simulink model "Simulare_Hrenciuc_Alexandru_motor_Petrom"  (R2018b)
settings: Solver=FixedStepAuto  StartTime=0.0  StopTime=0.2  FixedStep=0.00001  RelTol=1e-3
libraries: powerlib x19, powerlib_meascontrol x1, simulink x1
settings Model: Creator=alexa  LastModifiedBy=alexa

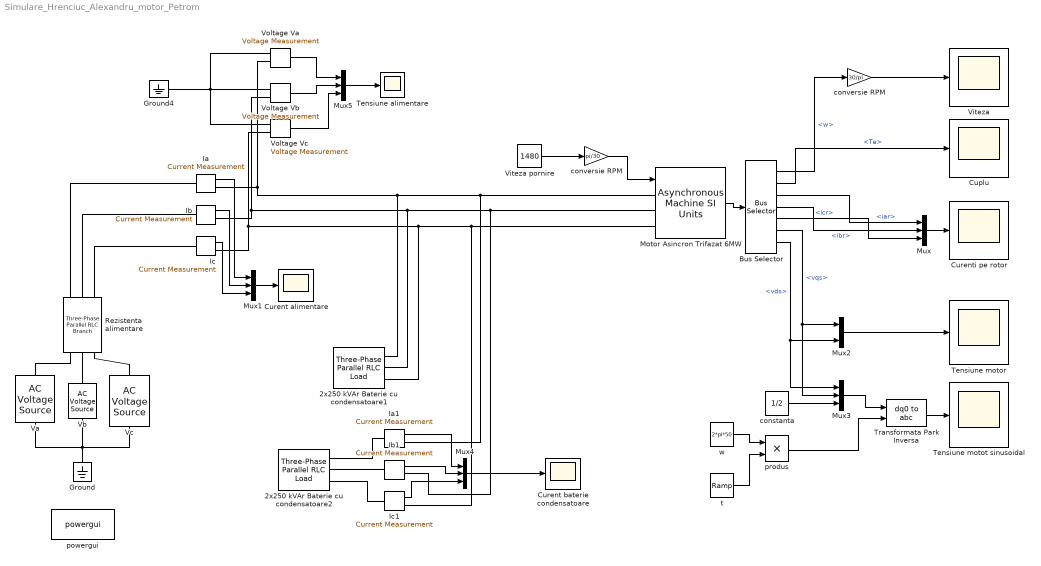
== system Simulare_Hrenciuc_Alexandru_motor_Petrom ==
  2x250 kVAr Baterie cu condensatoare1 : powerlib/Elements/Three-Phase Parallel RLC Load  LConnTagsString=A|B|C  Configuration=Delta  NominalVoltage=6000  Vabc=[1e3 1e3 1e3]  Vabcp=[1e3 1e3 1e3]  NominalFrequency=50  UnbalancedPower=off  ActivePower=0  InductivePower=0  CapacitivePower=5000000  Pabc=[10e3 9e3 11e3]  QLabc=[100 90 110]  QCabc=[100 90 110]  Pabcp=[10e3 9e3 11e3]  QLabcp=[100 90 110]  QCabcp=[100 90 110]  Measurements=Branch currents  LoadType=constant I
  2x250 kVAr Baterie cu condensatoare2 : powerlib/Elements/Three-Phase Parallel RLC Load  LConnTagsString=A|B|C  Configuration=Delta  NominalVoltage=6000  Vabc=[1e3 1e3 1e3]  Vabcp=[1e3 1e3 1e3]  NominalFrequency=50  UnbalancedPower=off  ActivePower=0  InductivePower=0  CapacitivePower=500000  Pabc=[10e3 9e3 11e3]  QLabc=[100 90 110]  QCabc=[100 90 110]  Pabcp=[0 0 0]  QLabcp=[0 0 0]  QCabcp=[1000 900 1100]  Measurements=Branch currents  LoadType=constant I
  Bus Selector : BusSelector  OutputSignals=w,Te,iar,ibr,icr,vqs,vds
  Cuplu : Scope
  Curent alimentare : Scope
  Curent baterie condensatoare : Scope
  Curenti pe rotor : Scope
  Ground : powerlib/Elements/Ground  LConnTagsString=a
  Ground4 : powerlib/Elements/Ground  LConnTagsString=a
  Ia : powerlib/Measurements/Current Measurement  PhasorSimulation=off  OutputType=Magnitude  PSBequivalent=0
  Ia1 : powerlib/Measurements/Current Measurement  PhasorSimulation=off  OutputType=Magnitude  PSBequivalent=0
  Ib : powerlib/Measurements/Current Measurement  PhasorSimulation=off  OutputType=Magnitude  PSBequivalent=0
  Ib1 : powerlib/Measurements/Current Measurement  PhasorSimulation=off  OutputType=Magnitude  PSBequivalent=0
  Ic : powerlib/Measurements/Current Measurement  PhasorSimulation=off  OutputType=Magnitude  PSBequivalent=0
  Ic1 : powerlib/Measurements/Current Measurement  PhasorSimulation=off  OutputType=Magnitude  PSBequivalent=0
  Motor Asincron Trifazat 6MW : powerlib/Machines/Asynchronous Machine SI Units  RotorType=Squirrel-cage  PresetModel=No  MechanicalLoad=Speed w  ShowDetailedParameters=on  ReferenceFrame=Synchronous  Units=SI  MeasurementBus=on  NominalParameters=[6.714e+06 6000 50]  Stator=[0.4 0.00064339]  Rotor=[0.82 0.00064339]  Cage1=[0.4155 0.002066]  Cage2=[0.4168 0.0003495]  Lm=0.0134  Mechanical=[330 0.005879 2]  PolePairs=2  InitialConditions=[0 0 0 0 0 0 0 0]  SimulateSaturation=off  Saturation=[14.03593122, 27.81365428, 53.79336849, 72.68890987, 97.98006896, 148.6815601, 215.7428561, 302.9841135, 428.7778367 ; 230, 322, 414, 460, 506, 552, 598, 644, 690]  LoadFlowParameters=1492000  TsPowergui=0  TsBlock=-1  IterativeModel=Trapezoidal non iterative  IterativeDiscreteModel=Trapezoidal non iterative  Pmec=6714000
  Mux{,1,3..5} (5 alike) : Mux  Inputs=3
  Mux2 : Mux  Inputs=2
  Rezistenta alimentare : powerlib/Elements/Three-Phase Parallel RLC Branch  LConnTagsString=A|B|C  RConnTagsString=A|B|C  BranchType=R  Resistance=0.95  Inductance=1e-3  Capacitance=1e-6  Measurements=None
      settings: SourceProductName=Simscape Power Systems  SourceProductBaseCode=PS
  Tensiune alimentare : Scope
  Tensiune motor : Scope
  Tensiune motot sinusoidal : Scope
  Transformata Park Inversa : powerlib_meascontrol/Transformations/dq0 to abc  Alignment=90 degrees behind phase A axis
  Va : powerlib/Electrical Sources/AC Voltage Source  Amplitude=4899  Phase=0  Frequency=50  SampleTime=0  Measurements=None  BusType=swing  Pref=10e3  Qref=0  Qmin=-inf  Qmax=+inf
  "Vb " : powerlib/Electrical Sources/AC Voltage Source  Amplitude=4899  Phase=-120  Frequency=50  SampleTime=0  Measurements=None  BusType=swing  Pref=10e3  Qref=0  Qmin=-inf  Qmax=+inf
  Vc : powerlib/Electrical Sources/AC Voltage Source  Amplitude=4899  Phase=120  Frequency=50  SampleTime=0  Measurements=None  BusType=swing  Pref=10e3  Qref=0  Qmin=-inf  Qmax=+inf
  Viteza : Scope
  Viteza pornire : Constant  Value=1480
  Voltage Va : powerlib/Measurements/Voltage Measurement  PhasorSimulation=off  OutputType=Complex  PSBequivalent=0
  Voltage Vb : powerlib/Measurements/Voltage Measurement  PhasorSimulation=off  OutputType=Complex  PSBequivalent=0
  Voltage Vc : powerlib/Measurements/Voltage Measurement  PhasorSimulation=off  OutputType=Complex  PSBequivalent=0
  "constanta " : Constant  Value=1/2
  conversie RPM : Gain  Gain=30/pi  SaturateOnIntegerOverflow=on  OutDataTypeStr=Inherit: Same as input  ParamDataTypeStr=Inherit: Same as input
  "conversie RPM " : Gain  Gain=pi/30  SaturateOnIntegerOverflow=on  OutDataTypeStr=Inherit: Same as input  ParamDataTypeStr=Inherit: Same as input
  powergui : powerlib/powergui  Priority=1  SimulationMode=Discrete  SampleTime=50e-6  frequency=50  Iterations=50  frequencyindice=50  Pbase=100e6  ErrMax=1e-4  UnitsV=kV  UnitsW=MW  buscounter=0  FunctionMessages=off  echomessages=off  EnableUseOfTLC=off  CurrentSourceSwitches=off  DisableSnubberDevices=off  DisableRonSwitches=off  DisableVfSwitches=off  DisplayEquations=off  SolverType=Tustin/Backward Euler (TBE)  Interpol=off  ExternalGateDelay=off  methode=off  Ts=100  x0status=blocks  SPID=off  SwTol=0  HookPort=off  RestoreLinks=warning  ResistiveCurrentMeasurement=off  Frange=[0:2:500]  Ylog=off  Xlog=on  ShowGrid=off  save=off  variable=ZData  structure=0  ZoomFFT=off  StartTime=0.0  cycles=1  DisplayStyle=1  fundamental=60  FreqAxis=off  MaxFrequency=1000  frequencyindicesteady=1  RmsSteady=1  display=off
  produs : Product  Inputs=**
  t : simulink/Sources/Ramp  slope=1  start=0  InitialOutput=0
  w : Constant  Value=2*pi*50
  wires:
  conversie RPM/1 -> Viteza/1
  Bus Selector/1 -> conversie RPM/1  "<w>"
  Motor Asincron Trifazat 6MW/1 -> Bus Selector/1
  Mux/1 -> Curenti pe rotor/1
  Ia/1 -> Mux1/1
  Ib/1 -> Mux1/2
  Ic/1 -> Mux1/3
  Mux1/1 -> Curent alimentare/1
  Transformata Park Inversa/1 -> Tensiune motot sinusoidal/1
  w/1 -> produs/1
  t/1 -> produs/2
  produs/1 -> Transformata Park Inversa/2
  Mux3/1 -> Transformata Park Inversa/1
  "constanta "/1 -> Mux3/3
  Mux2/1 -> Tensiune motor/1
  Ia1/1 -> Mux4/1
  Ib1/1 -> Mux4/2
  Ic1/1 -> Mux4/3
  Mux4/1 -> Curent baterie condensatoare/1
  Bus Selector/2 -> Cuplu/1  "<Te>"
  Bus Selector/3 -> Mux/1  "<iar>"
  Bus Selector/4 -> Mux/2  "<ibr>"
  Bus Selector/5 -> Mux/3  "<icr>"
  Bus Selector/6 -> Mux3/2, Mux2/1  "<vqs>"
  Bus Selector/7 -> Mux3/1, Mux2/2  "<vds>"
  Viteza pornire/1 -> "conversie RPM "/1
  "conversie RPM "/1 -> Motor Asincron Trifazat 6MW/1
  Mux5/1 -> Tensiune alimentare/1
  Voltage Va/1 -> Mux5/1
  Voltage Vb/1 -> Mux5/2
  Voltage Vc/1 -> Mux5/3
  connections:
  Va/LConn1 -- "Vb "/LConn1 -- Ground/LConn1 -- Vc/LConn1
  Ib/RConn1 -- Voltage Vb/LConn2 -- Ib1/RConn1 -- Motor Asincron Trifazat 6MW/LConn2 -- 2x250 kVAr Baterie cu condensatoare1/LConn2
  Ic/RConn1 -- Voltage Vc/LConn2 -- Motor Asincron Trifazat 6MW/LConn3 -- Ic1/RConn1 -- 2x250 kVAr Baterie cu condensatoare1/LConn3
  Va/RConn1 -- Rezistenta alimentare/LConn1
  "Vb "/RConn1 -- Rezistenta alimentare/LConn2
  Vc/RConn1 -- Rezistenta alimentare/LConn3
  Rezistenta alimentare/RConn1 -- Ia/LConn1
  Rezistenta alimentare/RConn2 -- Ib/LConn1
  Rezistenta alimentare/RConn3 -- Ic/LConn1
  Ia1/LConn1 -- 2x250 kVAr Baterie cu condensatoare2/LConn1
  Ib1/LConn1 -- 2x250 kVAr Baterie cu condensatoare2/LConn2
  Ic1/LConn1 -- 2x250 kVAr Baterie cu condensatoare2/LConn3
  Ia/RConn1 -- Voltage Va/LConn2 -- Ia1/RConn1 -- Motor Asincron Trifazat 6MW/LConn1 -- 2x250 kVAr Baterie cu condensatoare1/LConn1
  Ground4/LConn1 -- Voltage Vc/LConn1 -- Voltage Vb/LConn1 -- Voltage Va/LConn1
